simulink model "sin1pha"  (R2022b)
settings: Solver=VariableStepAuto  StartTime=0.0  StopTime=0.03  RelTol=1e-3
libraries: spsIGBTLib x4, simulink x2, spsDCVoltageSourceLib x1, spsTriangleGeneratorLib x1, spsVoltageMeasurementLib x1, sps_lib x1
settings Model: Creator=doand  LastModifiedBy=doand

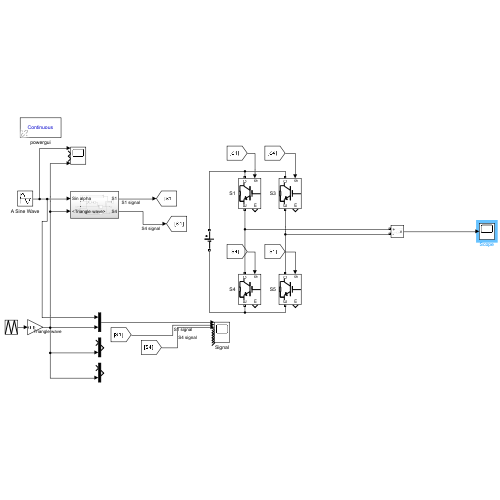
[thumbnail: Simulink's stored preview of the top-level diagram]
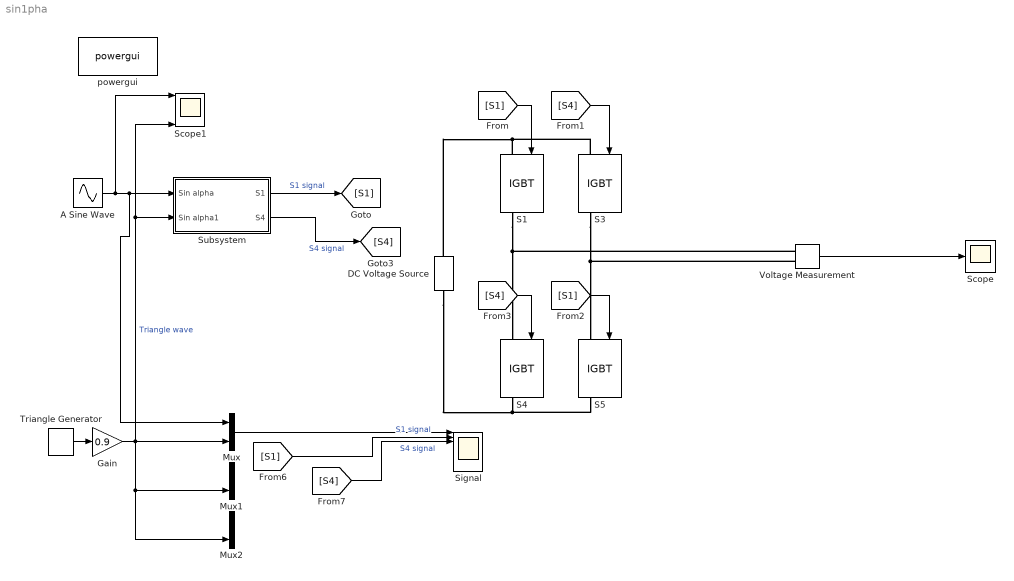
== system sin1pha ==
  A Sine Wave : Sin  Frequency=2*pi*50  SampleTime=0
  DC Voltage Source : spsDCVoltageSourceLib/DC Voltage Source  Amplitude=600  Measurements=None
  Gain : Gain  Gain=0.9
  Mux : Mux  Inputs=2
  Mux1 : Mux  Inputs=2
  Mux2 : Mux  Inputs=2
  S{1,3..5} (4 alike) : spsIGBTLib/IGBT  Ron=0.001  Lon=0  Vf=1  Tf=1e-6  Tt=2e-6  IC=0  Rs=1e5  Cs=inf  Measurements=on
  Scope : Scope
  Scope1 : Scope  NumInputPorts=4
  Signal : Scope  NumInputPorts=9
  Subsystem : Subsystem
  Triangle Generator : spsTriangleGeneratorLib/Triangle Generator  Freq=2000*4  Phase=0  Ts=0
  Voltage Measurement : spsVoltageMeasurementLib/Voltage Measurement  PhasorSimulation=off  OutputType=Complex  PSBequivalent=0
  powergui : sps_lib/powergui  Priority=1  SimulationMode=Continuous  SampleTime=50e-6  frequency=60  Iterations=50  frequencyindice=0  Pbase=100e6  ErrMax=1e-4  UnitsV=kV  UnitsW=MW  buscounter=0  FunctionMessages=off  echomessages=off  EnableUseOfTLC=off  CurrentSourceSwitches=off  DisableSnubberDevices=off  DisableRonSwitches=off  DisableVfSwitches=off  DisplayEquations=off  AutomaticDiscreteSolvers=off  SolverType=Tustin/Backward Euler (TBE)  Interpol=off  ExternalGateDelay=off  methode=off  Ts=100  x0status=blocks  SPID=on  SwTol=0  HookPort=off  NonlinearTolerance=1e-4  nMaxIteration=100  ContinueOnMaxIteration=off  RestoreLinks=warning  ResistiveCurrentMeasurement=off  Frange=[0:2:500]  Ylog=off  Xlog=on  ShowGrid=off  save=off  variable=ZData  structure=0  ZoomFFT=off  StartTime=0.0  cycles=1  DisplayStyle=1  fundamental=60  FreqAxis=off  MaxFrequency=1000  frequencyindicesteady=1  RmsSteady=1  display=off
  wires:
  Mux/1 -> Signal/1
  [S4] -> S4/1
  [S4] -> Signal/3  "S4 signal"
  Triangle Generator/1 -> Gain/1
  [S1] -> S1/1
  [S1] -> Signal/2  "S1 signal"
  A Sine Wave/1 -> Scope1/1, Subsystem/1(Sin alpha), Mux/1
  Gain/1 -> Scope1/4, Subsystem/2(Sin alpha1), Mux2/2, Mux1/2, Mux/2  "Triangle wave"
  [S4] -> S3/1
  Subsystem/2(S4) -> [S4]  "S4 signal"
  [S1] -> S5/1
  Subsystem/1(S1) -> [S1]  "S1 signal"
  Voltage Measurement/1 -> Scope/1
  connections:
  S3/RConn1 -- S5/LConn1 -- Voltage Measurement/LConn2
  S3/LConn1 -- DC Voltage Source/RConn1 -- S1/LConn1
  S5/RConn1 -- DC Voltage Source/LConn1 -- S4/RConn1
  S1/RConn1 -- S4/LConn1 -- Voltage Measurement/LConn1

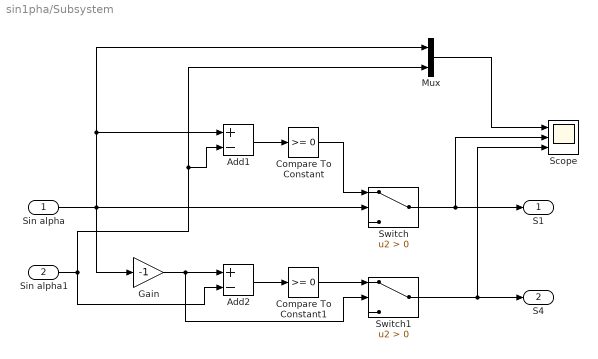
== system sin1pha/Subsystem ==
  Sin alpha : Inport
  Sin alpha1 : Inport  Port=2
  Add1 : Sum  Inputs=+-
  Add2 : Sum  Inputs=+-
  Compare To Constant : simulink/Logic and Bit Operations/Compare To Constant  relop=>=  const=0  OutDataTypeStr=boolean
  Compare To Constant1 : simulink/Logic and Bit Operations/Compare To Constant  relop=>=  const=0  OutDataTypeStr=boolean
  Gain : Gain  Gain=-1
  Mux : Mux  Inputs=2
  Scope : Scope  NumInputPorts=3
  Switch : Switch  Criteria=u2 > Threshold  SaturateOnIntegerOverflow=off  InputSameDT=off
  Switch1 : Switch  Criteria=u2 > Threshold  SaturateOnIntegerOverflow=off  InputSameDT=off
  S1 : Outport
  S4 : Outport  Port=2
  wires:
  Sin alpha/1 -> Gain/1, Switch/2, Mux/1, Add1/1
  Add1/1 -> Compare To Constant/1
  Compare To Constant/1 -> Switch/1
  Switch/1 -> Scope/2, S1/1
  Switch1/1 -> Scope/3, S4/1
  Sin alpha1/1 -> Add2/2, Mux/2, Add1/2
  Add2/1 -> Compare To Constant1/1
  Gain/1 -> Switch1/2, Add2/1
  Compare To Constant1/1 -> Switch1/1
  Mux/1 -> Scope/1
